simulink model "SM_Offshore_Windturbine"  (R2021a)
settings: Solver=ode4  StartTime=0.0  StopTime=par.sym.Ttot  FixedStep=par.sym.max_dt  MaxStep=par.sym.max_dt  RelTol=1e-3
model workspace: external: MATLAB File C:\Users\d053704\Desktop\MOST\Structure\CAD\CAD_DataFile.m (data not in the file)
undefined symbols (not defined in the file): par, smiData, X, Y, Z
libraries: sm_lib x50, simulink_extras x29, vrlib x18, nesl_utility x10, dspstat3 x9, sharedutil x5, eeGeneralControl x2
(part 2 of 4)

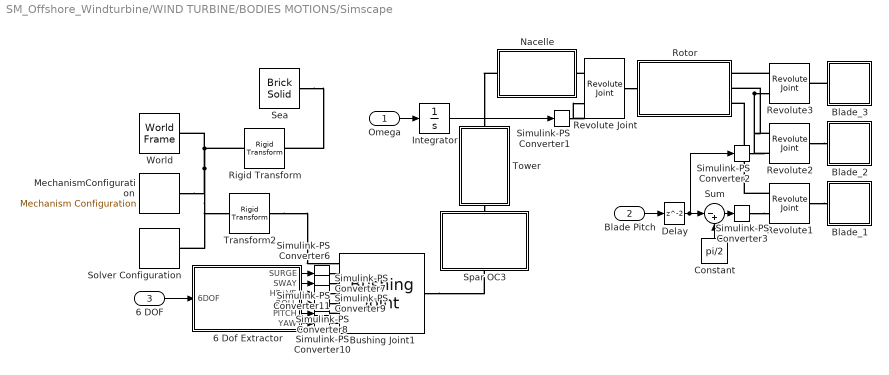
== system SM_Offshore_Windturbine/WIND TURBINE/BODIES MOTIONS/Simscape ==
  Omega : Inport
  Blade Pitch : Inport  Port=2
  6 DOF : Inport  Port=3
  "6 Dof Extractor " : Subsystem
  Blade_1 : Subsystem
  Blade_2 : Subsystem
  Blade_3 : Subsystem
  Bushing Joint1 : sm_lib/Joints/Bushing Joint  JointMode=Normal  SenseConstraintForce=off  SenseConstraintForceX=off  SenseConstraintForceY=off  SenseConstraintForceZ=off  SenseConstraintTorque=off  SenseConstraintTorqueX=off  SenseConstraintTorqueY=off  SenseConstraintTorqueZ=off  SenseTotalForce=off  SenseTotalForceX=off  SenseTotalForceY=off  SenseTotalForceZ=off  SenseTotalTorque=off  SenseTotalTorqueX=off  SenseTotalTorqueY=off  SenseTotalTorqueZ=off  CompositeWrenchDir=FollowerOnBase  CompositeWrenchFrame=BaseFrame  PxEquilibriumPosition=0  PxEquilibriumPositionUnits=m  PxSpringStiffness=0  PxSpringStiffnessUnits=N/m  PxDampingCoefficient=0  PxDampingCoefficientUnits=N/(m/s)  PxTorqueActuationMode=ComputedTorque  PxMotionActuationMode=InputMotion  PxSensePosition=off  PxSenseVelocity=off  PxSenseAcceleration=off  PxSenseTorqueForce=off  PxSenseLowerLimitTorqueForce=off  PxSenseUpperLimitTorqueForce=off  PxLowerLimitSpecify=off  PxLowerLimitBound=-1  PxLowerLimitBoundUnits=m  PxLowerLimitStiffness=1e6  PxLowerLimitStiffnessUnits=N/m  PxLowerLimitDamping=1e3  PxLowerLimitDampingUnits=N/(m/s)  PxLowerLimitTransitionRegionWidth=1e-4  PxLowerLimitTransitionRegionWidthUnits=m  PxUpperLimitSpecify=off  PxUpperLimitBound=1  PxUpperLimitBoundUnits=m  PxUpperLimitStiffness=1e6  PxUpperLimitStiffnessUnits=N/m  PxUpperLimitDamping=1e3  PxUpperLimitDampingUnits=N/(m/s)  PxUpperLimitTransitionRegionWidth=1e-4  PxUpperLimitTransitionRegionWidthUnits=m  PxPositionTargetSpecify=off  PxPositionTargetPriority=High  PxPositionTargetValue=0  PxPositionTargetValueUnits=m  PxVelocityTargetSpecify=off  PxVelocityTargetPriority=High  PxVelocityTargetValue=0  PxVelocityTargetValueUnits=m/s  PyEquilibriumPosition=0  PyEquilibriumPositionUnits=m  PySpringStiffness=0  PySpringStiffnessUnits=N/m  PyDampingCoefficient=0  PyDampingCoefficientUnits=N/(m/s)  PyTorqueActuationMode=ComputedTorque  PyMotionActuationMode=InputMotion  PySensePosition=off  PySenseVelocity=off  PySenseAcceleration=off  PySenseTorqueForce=off  PySenseLowerLimitTorqueForce=off  PySenseUpperLimitTorqueForce=off  PyLowerLimitSpecify=off  PyLowerLimitBound=-1  PyLowerLimitBoundUnits=m  PyLowerLimitStiffness=1e6  PyLowerLimitStiffnessUnits=N/m  PyLowerLimitDamping=1e3  PyLowerLimitDampingUnits=N/(m/s)  PyLowerLimitTransitionRegionWidth=1e-4  PyLowerLimitTransitionRegionWidthUnits=m  PyUpperLimitSpecify=off  PyUpperLimitBound=1  PyUpperLimitBoundUnits=m  PyUpperLimitStiffness=1e6  PyUpperLimitStiffnessUnits=N/m  PyUpperLimitDamping=1e3  PyUpperLimitDampingUnits=N/(m/s)  PyUpperLimitTransitionRegionWidth=1e-4  PyUpperLimitTransitionRegionWidthUnits=m  PyPositionTargetSpecify=off  PyPositionTargetPriority=High  PyPositionTargetValue=0  PyPositionTargetValueUnits=m  PyVelocityTargetSpecify=off  PyVelocityTargetPriority=High  PyVelocityTargetValue=0  PyVelocityTargetValueUnits=m/s  PzEquilibriumPosition=0  PzEquilibriumPositionUnits=m  PzSpringStiffness=0  PzSpringStiffnessUnits=N/m  PzDampingCoefficient=0  PzDampingCoefficientUnits=N/(m/s)  PzTorqueActuationMode=ComputedTorque  PzMotionActuationMode=InputMotion  PzSensePosition=off  PzSenseVelocity=off  PzSenseAcceleration=off  PzSenseTorqueForce=off  PzSenseLowerLimitTorqueForce=off  PzSenseUpperLimitTorqueForce=off  PzLowerLimitSpecify=off  PzLowerLimitBound=-1  PzLowerLimitBoundUnits=m  PzLowerLimitStiffness=1e6  PzLowerLimitStiffnessUnits=N/m  PzLowerLimitDamping=1e3  PzLowerLimitDampingUnits=N/(m/s)  PzLowerLimitTransitionRegionWidth=1e-4  PzLowerLimitTransitionRegionWidthUnits=m  PzUpperLimitSpecify=off  PzUpperLimitBound=1  PzUpperLimitBoundUnits=m  PzUpperLimitStiffness=1e6  PzUpperLimitStiffnessUnits=N/m  PzUpperLimitDamping=1e3  PzUpperLimitDampingUnits=N/(m/s)  PzUpperLimitTransitionRegionWidth=1e-4  PzUpperLimitTransitionRegionWidthUnits=m  PzPositionTargetSpecify=off  PzPositionTargetPriority=High  PzPositionTargetValue=0  PzPositionTargetValueUnits=m  PzVelocityTargetSpecify=off  PzVelocityTargetPriority=High  PzVelocityTargetValue=0  PzVelocityTargetValueUnits=m/s  RxEquilibriumPosition=0  RxEquilibriumPositionUnits=deg  RxSpringStiffness=0  RxSpringStiffnessUnits=N*m/deg  RxDampingCoefficient=0  RxDampingCoefficientUnits=N*m/(deg/s)  RxTorqueActuationMode=ComputedTorque  RxMotionActuationMode=InputMotion  RxSensePosition=off  RxSenseVelocity=off  RxSenseAcceleration=off  RxSenseTorqueForce=off  RxSenseLowerLimitTorqueForce=off  RxSenseUpperLimitTorqueForce=off  RxLowerLimitSpecify=off  RxLowerLimitBound=-90  RxLowerLimitBoundUnits=deg  RxLowerLimitStiffness=1e4  RxLowerLimitStiffnessUnits=N*m/deg  RxLowerLimitDamping=10  RxLowerLimitDampingUnits=N*m/(deg/s)  RxLowerLimitTransitionRegionWidth=0.1  RxLowerLimitTransitionRegionWidthUnits=deg  RxUpperLimitSpecify=off  RxUpperLimitBound=90  RxUpperLimitBoundUnits=deg  RxUpperLimitStiffness=1e4  RxUpperLimitStiffnessUnits=N*m/deg  RxUpperLimitDamping=10  RxUpperLimitDampingUnits=N*m/(deg/s)  RxUpperLimitTransitionRegionWidth=0.1  RxUpperLimitTransitionRegionWidthUnits=deg  RxPositionTargetSpecify=off  RxPositionTargetPriority=High  RxPositionTargetValue=0  RxPositionTargetValueUnits=deg  RxVelocityTargetSpecify=off  RxVelocityTargetPriority=High  RxVelocityTargetValue=0  RxVelocityTargetValueUnits=deg/s  RyEquilibriumPosition=0  RyEquilibriumPositionUnits=deg  RySpringStiffness=0  RySpringStiffnessUnits=N*m/deg  RyDampingCoefficient=0  RyDampingCoefficientUnits=N*m/(deg/s)  RyTorqueActuationMode=ComputedTorque  RyMotionActuationMode=InputMotion  RySensePosition=off  RySenseVelocity=off  RySenseAcceleration=off  RySenseTorqueForce=off  RySenseLowerLimitTorqueForce=off  RySenseUpperLimitTorqueForce=off  RyLowerLimitSpecify=off  RyLowerLimitBound=-90  RyLowerLimitBoundUnits=deg  RyLowerLimitStiffness=1e4  RyLowerLimitStiffnessUnits=N*m/deg  RyLowerLimitDamping=10  RyLowerLimitDampingUnits=N*m/(deg/s)  RyLowerLimitTransitionRegionWidth=0.1  RyLowerLimitTransitionRegionWidthUnits=deg  RyUpperLimitSpecify=off  RyUpperLimitBound=90  RyUpperLimitBoundUnits=deg  RyUpperLimitStiffness=1e4  RyUpperLimitStiffnessUnits=N*m/deg  RyUpperLimitDamping=10  RyUpperLimitDampingUnits=N*m/(deg/s)  RyUpperLimitTransitionRegionWidth=0.1  RyUpperLimitTransitionRegionWidthUnits=deg  RyPositionTargetSpecify=off  RyPositionTargetPriority=High  RyPositionTargetValue=0  RyPositionTargetValueUnits=deg  RyVelocityTargetSpecify=off  RyVelocityTargetPriority=High  RyVelocityTargetValue=0  RyVelocityTargetValueUnits=deg/s  RzEquilibriumPosition=0  RzEquilibriumPositionUnits=deg  RzSpringStiffness=0  RzSpringStiffnessUnits=N*m/deg  RzDampingCoefficient=0  RzDampingCoefficientUnits=N*m/(deg/s)  RzTorqueActuationMode=ComputedTorque  RzMotionActuationMode=InputMotion  RzSensePosition=off  RzSenseVelocity=off  RzSenseAcceleration=off  RzSenseTorqueForce=off  RzSenseLowerLimitTorqueForce=off  RzSenseUpperLimitTorqueForce=off  RzLowerLimitSpecify=off  RzLowerLimitBound=-90  RzLowerLimitBoundUnits=deg  RzLowerLimitStiffness=1e4  RzLowerLimitStiffnessUnits=N*m/deg  RzLowerLimitDamping=10  RzLowerLimitDampingUnits=N*m/(deg/s)  RzLowerLimitTransitionRegionWidth=0.1  RzLowerLimitTransitionRegionWidthUnits=deg  RzUpperLimitSpecify=off  RzUpperLimitBound=90  RzUpperLimitBoundUnits=deg  RzUpperLimitStiffness=1e4  RzUpperLimitStiffnessUnits=N*m/deg  RzUpperLimitDamping=10  RzUpperLimitDampingUnits=N*m/(deg/s)  RzUpperLimitTransitionRegionWidth=0.1  RzUpperLimitTransitionRegionWidthUnits=deg  RzPositionTargetSpecify=off  RzPositionTargetPriority=High  RzPositionTargetValue=0  RzPositionTargetValueUnits=deg  RzVelocityTargetSpecify=off  RzVelocityTargetPriority=High  RzVelocityTargetValue=0  RzVelocityTargetValueUnits=deg/s
  Constant : Constant  Value=pi/2
  Delay : Delay
  Integrator : Integrator
  MechanismConfiguration : sm_lib/Utilities/Mechanism Configuration  UniformGravity=Constant  GravityVector=[0 -9.80665 0]  GravityVectorUnits=m/s^2  GravityUnits=m/s^2  LinearizationDelta=0.001  JointModeTransitionNonlinearIterations=2
  Nacelle : Subsystem
  Revolute Joint : sm_lib/Joints/Revolute Joint  JointMode=Normal  SenseConstraintForce=off  SenseConstraintForceX=off  SenseConstraintForceY=off  SenseConstraintForceZ=off  SenseConstraintTorque=off  SenseConstraintTorqueX=off  SenseConstraintTorqueY=off  SenseConstraintTorqueZ=off  SenseTotalForce=off  SenseTotalForceX=off  SenseTotalForceY=off  SenseTotalForceZ=off  SenseTotalTorque=off  SenseTotalTorqueX=off  SenseTotalTorqueY=off  SenseTotalTorqueZ=off  CompositeWrenchDir=FollowerOnBase  CompositeWrenchFrame=BaseFrame  EquilibriumPosition=0  EquilibriumPositionUnits=deg  SpringStiffness=0  SpringStiffnessUnits=N*m/deg  DampingCoefficient=0  DampingCoefficientUnits=N*m/(rad/s)  TorqueActuationMode=ComputedTorque  MotionActuationMode=InputMotion  SensePosition=off  SenseVelocity=off  SenseAcceleration=off  SenseTorqueForce=off  SenseLowerLimitTorqueForce=off  SenseUpperLimitTorqueForce=off  LowerLimitSpecify=off  LowerLimitBound=-90  LowerLimitBoundUnits=deg  LowerLimitStiffness=1e4  LowerLimitStiffnessUnits=N*m/deg  LowerLimitDamping=10  LowerLimitDampingUnits=N*m/(deg/s)  LowerLimitTransitionRegionWidth=0.1  LowerLimitTransitionRegionWidthUnits=deg  UpperLimitSpecify=off  UpperLimitBound=90  UpperLimitBoundUnits=deg  UpperLimitStiffness=1e4  UpperLimitStiffnessUnits=N*m/deg  UpperLimitDamping=10  UpperLimitDampingUnits=N*m/(deg/s)  UpperLimitTransitionRegionWidth=0.1  UpperLimitTransitionRegionWidthUnits=deg  PositionTargetSpecify=on  PositionTargetPriority=High  PositionTargetValue=0  PositionTargetValueUnits=deg  VelocityTargetSpecify=on  VelocityTargetPriority=High  VelocityTargetValue=12.1/60  VelocityTargetValueUnits=rev/s
  Revolute1 : sm_lib/Joints/Revolute Joint  JointMode=Normal  SenseConstraintForce=off  SenseConstraintForceX=off  SenseConstraintForceY=off  SenseConstraintForceZ=off  SenseConstraintTorque=off  SenseConstraintTorqueX=off  SenseConstraintTorqueY=off  SenseConstraintTorqueZ=off  SenseTotalForce=off  SenseTotalForceX=off  SenseTotalForceY=off  SenseTotalForceZ=off  SenseTotalTorque=off  SenseTotalTorqueX=off  SenseTotalTorqueY=off  SenseTotalTorqueZ=off  CompositeWrenchDir=FollowerOnBase  CompositeWrenchFrame=BaseFrame  EquilibriumPosition=0  EquilibriumPositionUnits=rad  SpringStiffness=0  SpringStiffnessUnits=N*m/rad  DampingCoefficient=0  DampingCoefficientUnits=N*m/(rad/s)  TorqueActuationMode=ComputedTorque  MotionActuationMode=InputMotion  SensePosition=off  SenseVelocity=off  SenseAcceleration=off  SenseTorqueForce=off  SenseLowerLimitTorqueForce=off  SenseUpperLimitTorqueForce=off  LowerLimitSpecify=off  LowerLimitBound=-90  LowerLimitBoundUnits=deg  LowerLimitStiffness=1e4  LowerLimitStiffnessUnits=N*m/deg  LowerLimitDamping=10  LowerLimitDampingUnits=N*m/(deg/s)  LowerLimitTransitionRegionWidth=0.1  LowerLimitTransitionRegionWidthUnits=deg  UpperLimitSpecify=off  UpperLimitBound=90  UpperLimitBoundUnits=deg  UpperLimitStiffness=1e4  UpperLimitStiffnessUnits=N*m/deg  UpperLimitDamping=10  UpperLimitDampingUnits=N*m/(deg/s)  UpperLimitTransitionRegionWidth=0.1  UpperLimitTransitionRegionWidthUnits=deg  PositionTargetSpecify=on  PositionTargetPriority=High  PositionTargetValue=90  PositionTargetValueUnits=deg  VelocityTargetSpecify=off  VelocityTargetPriority=High  VelocityTargetValue=0  VelocityTargetValueUnits=deg/s
  Revolute2 : sm_lib/Joints/Revolute Joint  JointMode=Normal  SenseConstraintForce=off  SenseConstraintForceX=off  SenseConstraintForceY=off  SenseConstraintForceZ=off  SenseConstraintTorque=off  SenseConstraintTorqueX=off  SenseConstraintTorqueY=off  SenseConstraintTorqueZ=off  SenseTotalForce=off  SenseTotalForceX=off  SenseTotalForceY=off  SenseTotalForceZ=off  SenseTotalTorque=off  SenseTotalTorqueX=off  SenseTotalTorqueY=off  SenseTotalTorqueZ=off  CompositeWrenchDir=FollowerOnBase  CompositeWrenchFrame=BaseFrame  EquilibriumPosition=0  EquilibriumPositionUnits=rad  SpringStiffness=0  SpringStiffnessUnits=N*m/rad  DampingCoefficient=0  DampingCoefficientUnits=N*m/(rad/s)  TorqueActuationMode=ComputedTorque  MotionActuationMode=InputMotion  SensePosition=off  SenseVelocity=off  SenseAcceleration=off  SenseTorqueForce=off  SenseLowerLimitTorqueForce=off  SenseUpperLimitTorqueForce=off  LowerLimitSpecify=off  LowerLimitBound=-90  LowerLimitBoundUnits=deg  LowerLimitStiffness=1e4  LowerLimitStiffnessUnits=N*m/deg  LowerLimitDamping=10  LowerLimitDampingUnits=N*m/(deg/s)  LowerLimitTransitionRegionWidth=0.1  LowerLimitTransitionRegionWidthUnits=deg  UpperLimitSpecify=off  UpperLimitBound=90  UpperLimitBoundUnits=deg  UpperLimitStiffness=1e4  UpperLimitStiffnessUnits=N*m/deg  UpperLimitDamping=10  UpperLimitDampingUnits=N*m/(deg/s)  UpperLimitTransitionRegionWidth=0.1  UpperLimitTransitionRegionWidthUnits=deg  PositionTargetSpecify=on  PositionTargetPriority=High  PositionTargetValue=0  PositionTargetValueUnits=deg  VelocityTargetSpecify=off  VelocityTargetPriority=High  VelocityTargetValue=0  VelocityTargetValueUnits=deg/s
  Revolute3 : sm_lib/Joints/Revolute Joint  JointMode=Normal  SenseConstraintForce=off  SenseConstraintForceX=off  SenseConstraintForceY=off  SenseConstraintForceZ=off  SenseConstraintTorque=off  SenseConstraintTorqueX=off  SenseConstraintTorqueY=off  SenseConstraintTorqueZ=off  SenseTotalForce=off  SenseTotalForceX=off  SenseTotalForceY=off  SenseTotalForceZ=off  SenseTotalTorque=off  SenseTotalTorqueX=off  SenseTotalTorqueY=off  SenseTotalTorqueZ=off  CompositeWrenchDir=FollowerOnBase  CompositeWrenchFrame=BaseFrame  EquilibriumPosition=0  EquilibriumPositionUnits=rad  SpringStiffness=0  SpringStiffnessUnits=N*m/rad  DampingCoefficient=0  DampingCoefficientUnits=N*m/(rad/s)  TorqueActuationMode=ComputedTorque  MotionActuationMode=InputMotion  SensePosition=off  SenseVelocity=off  SenseAcceleration=off  SenseTorqueForce=off  SenseLowerLimitTorqueForce=off  SenseUpperLimitTorqueForce=off  LowerLimitSpecify=off  LowerLimitBound=-90  LowerLimitBoundUnits=deg  LowerLimitStiffness=1e4  LowerLimitStiffnessUnits=N*m/deg  LowerLimitDamping=10  LowerLimitDampingUnits=N*m/(deg/s)  LowerLimitTransitionRegionWidth=0.1  LowerLimitTransitionRegionWidthUnits=deg  UpperLimitSpecify=off  UpperLimitBound=90  UpperLimitBoundUnits=deg  UpperLimitStiffness=1e4  UpperLimitStiffnessUnits=N*m/deg  UpperLimitDamping=10  UpperLimitDampingUnits=N*m/(deg/s)  UpperLimitTransitionRegionWidth=0.1  UpperLimitTransitionRegionWidthUnits=deg  PositionTargetSpecify=on  PositionTargetPriority=High  PositionTargetValue=0  PositionTargetValueUnits=deg  VelocityTargetSpecify=off  VelocityTargetPriority=High  VelocityTargetValue=0  VelocityTargetValueUnits=deg/s
  Rigid Transform : sm_lib/Frames and Transforms/Rigid Transform  TranslationMethod=Cartesian  TranslationStandardOffset=0  TranslationLengthUnit=m  TranslationStandardAxis=+Z  TranslationCartesianOffset=[-5 5 2]  TranslationROffset=0  TranslationROffsetUnits=m  TranslationZOffset=0  TranslationZOffsetUnits=m  TranslationThetaOffset=0  TranslationThetaOffsetUnits=deg  RotationMethod=None  RotationAngleUnits=deg  RotationStandardAxis=+Z  RotationAngle=0.0  RotationArbitraryAxis=[0 0 1]  FollAlignAxisA=+X  BaseAlignAxisA=+Y  FollAlignAxisB=+Y  BaseAlignAxisB=+Z  RotationSequenceAxes=FollowerAxes  RotationSequence=XYX  RotationSequenceAngles=[0 0 0]  RotationSequenceAnglesUnits=deg  RotationMatrix=[1 0 0; 0 1 0; 0 0 1]
  Rotor : Subsystem
  Sea : sm_lib/Body Elements/Brick Solid  GraphicAmbientColor=[0.15 0.15 0.15 1.0]  BasedOnType=Density  BrickDimensions=[300 300 1]  BrickDimensionUnits=m  CenterOfMass=[0 0 0]  CenterOfMassUnits=m  GraphicDiffuseColor=[0.0 0.79607844 1.0]  Density=1000  DensityUnits=kg/m^3  DoExposeReferenceFrame=on  GraphicEmissiveColor=[0.0 0.0 0.0 1.0]  ExportEntireGeometry=off  SerializedFrames=<Frames/>  MarkerShape=Sphere  MarkerSize=10  GraphicType=FromGeometry  InertiaType=CalculateFromGeometry  Mass=1  MassUnits=kg  MomentsOfInertia=[1 1 1]  MomentsOfInertiaUnits=kg*m^2  GraphicOpacity=0.5  ProductsOfInertia=[0 0 0]  ProductsOfInertiaUnits=kg*m^2  GraphicShininess=75  GraphicSpecularColor=[0.5 0.5 0.5 1.0]  GraphicVisPropType=SimpleVisualProperties
  Simulink-PS Converter{1..3,6..11} (9 alike) : nesl_utility/Simulink-PS Converter  PhysicalDomain=network_engine_domain  SubClassName=ps_input  LeftPortType=input  RightPortType=output  PseudoPeriodic=off  Frequencies=[]  NoiseDistribution=none  NoiseParameters=[]  Unit=1  AffineConversion=off  FilteringAndDerivatives=filter  SimscapeFilterOrder=2  InputFilterTimeConstant=0.05  UdotUserProvided=0
      settings: SourceProductBaseCode=PW,SS
  Solver Configuration : nesl_utility/Solver Configuration  PhysicalDomain=network_engine_domain  SubClassName=solver  LeftPortType=input  RightPortType=generic  Tones=[]  Harmonics=[]  SimulateNoise=off  Profile=off  UseLocalSampling=off  EnableSwitchedLinearOptims=on  FrequencyDomain=off  UseCCode=off  RelTol=0.001  AbsTol=1e-06  MinStep=1e-09  ToWorkspace=off  RevertToSquareIcSolve=off  NumHomotopyIterations=100  PhasorMode=off  PhasorModeNumHarmonics=1  DoDC=off  ResidualTolerance=1e-09  UseLocalSolver=off  LocalSolverChoice=NE_BACKWARD_EULER_ADVANCER  LocalSolverSampleTime=0.001  DoFixedCost=off  MaxNonlinIter=3  MaxModeIter=2  ComputeImpulses=off  ImpulseIterations=2  LinearAlgebra=auto  EquationFormulation=NE_TIME_EF  DelaysMemoryBudget=1024  AutomaticFiltering=on  FilteringTimeConstant=0.001  PartitionStorageMethod=AS_NEEDED  PartitionMemoryBudget=1024  PartitionMethod=FAST
      settings: SourceProductBaseCode=PW,SS
  Spar OC3 : Subsystem
  Sum : Sum  Inputs=|-+
  Tower : Subsystem
  Transform2 : sm_lib/Frames and Transforms/Rigid Transform  TranslationMethod=Cartesian  TranslationStandardOffset=0  TranslationLengthUnit=m  TranslationStandardAxis=+Z  TranslationCartesianOffset=smiData.RigidTransform(17).translation  TranslationROffset=0  TranslationROffsetUnits=m  TranslationZOffset=0  TranslationZOffsetUnits=m  TranslationThetaOffset=0  TranslationThetaOffsetUnits=deg  RotationMethod=ArbitraryAxis  RotationAngleUnits=rad  RotationStandardAxis=+Z  RotationAngle=smiData.RigidTransform(17).angle  RotationArbitraryAxis=smiData.RigidTransform(17).axis  FollAlignAxisA=+X  BaseAlignAxisA=+Y  FollAlignAxisB=+Y  BaseAlignAxisB=+Z  RotationSequenceAxes=FollowerAxes  RotationSequence=XYX  RotationSequenceAngles=[0 0 0]  RotationSequenceAnglesUnits=deg  RotationMatrix=[1 0 0; 0 1 0; 0 0 1]
  World : sm_lib/Frames and Transforms/World Frame
  wires:
  Integrator/1 -> Simulink-PS Converter1/1
  Blade Pitch/1 -> Delay/1
  "6 Dof Extractor "/1(SURGE) -> Simulink-PS Converter6/1
  "6 Dof Extractor "/6(YAW) -> Simulink-PS Converter11/1
  Sum/1 -> Simulink-PS Converter3/1
  Constant/1 -> Sum/2
  "6 Dof Extractor "/3(HEAVE) -> Simulink-PS Converter8/1
  "6 Dof Extractor "/5(PITCH) -> Simulink-PS Converter10/1
  "6 Dof Extractor "/4(ROLL) -> Simulink-PS Converter9/1
  6 DOF/1 -> "6 Dof Extractor "/1(6DOF)
  "6 Dof Extractor "/2(SWAY) -> Simulink-PS Converter7/1
  Delay/1 -> Simulink-PS Converter2/1, Sum/1
  Omega/1 -> Integrator/1
  connections:
  Revolute2/LConn1 -- Rotor/RConn2
  Simulink-PS Converter8/RConn1 -- Bushing Joint1/LConn4
  Revolute1/LConn1 -- Rotor/RConn3
  Simulink-PS Converter7/RConn1 -- Bushing Joint1/LConn3
  Nacelle/LConn1 -- Tower/RConn1
  Revolute2/RConn1 -- Blade_2/LConn1
  Simulink-PS Converter3/RConn1 -- Revolute1/LConn2
  Revolute Joint/LConn1 -- Nacelle/RConn1
  Revolute Joint/RConn1 -- Rotor/LConn1
  Transform2/RConn1 -- Bushing Joint1/LConn1
  Bushing Joint1/LConn6 -- Simulink-PS Converter10/RConn1
  Bushing Joint1/LConn7 -- Simulink-PS Converter11/RConn1
  Simulink-PS Converter6/RConn1 -- Bushing Joint1/LConn2
  Bushing Joint1/RConn1 -- Spar OC3/LConn1
  Revolute1/RConn1 -- Blade_1/LConn1
  Rigid Transform/LConn1 -- World/RConn1 -- MechanismConfiguration/RConn1 -- Solver Configuration/RConn1 -- Transform2/LConn1
  Simulink-PS Converter9/RConn1 -- Bushing Joint1/LConn5
  Revolute3/LConn1 -- Rotor/RConn1
  Simulink-PS Converter1/RConn1 -- Revolute Joint/LConn2
  Blade_3/LConn1 -- Revolute3/RConn1
  Revolute3/LConn2 -- Simulink-PS Converter2/RConn1 -- Revolute2/LConn2
  Tower/LConn1 -- Spar OC3/RConn1
  Sea/RConn1 -- Rigid Transform/RConn1

== system SM_Offshore_Windturbine/WIND TURBINE/CONTROL SYSTEM/BLADE PITCH CONTROL ==
  note: GK(theta)
  note: PITCH CONTROL
  Filtered generator speed : Inport
  Constant2 : Constant
  Constant3 : Constant
  Divide : Product  Inputs=*/
  Divide1 : Product  Inputs=*/
  Gain : Gain  Gain=pi/2
  Gain1 : Gain  Gain=par.WT.ctrl.PITCH.Kp_c
  Gain2 : Gain  Gain=par.WT.ctrl.PITCH.Ki_c
  Integrator Limited : Integrator  InitialCondition=par.IC.BlPtc0/180*pi / (par.WT.ctrl.PITCH.Ki_c / (1 + par.IC.BlPtc0/par.WT.ctrl.PITCH.thetak))  LimitOutput=on  LowerSaturationLimit=0
  Max : MinMax  Function=max  Inputs=2
  Memory : Memory  InitialCondition=par.IC.BlPtc0
  Min : MinMax  Inputs=2
  Pitch rate limiter : RateLimiter  RisingSlewLimit=par.WT.ctrl.PITCH.ratelim/180*pi  FallingSlewLimit=-par.WT.ctrl.PITCH.ratelim/180*pi  SampleTimeMode=inherited
  Pitch saturation : Saturate  UpperLimit=pi/2  LowerLimit=0
  Product : Product  RndMeth=Zero
  Product1 : Product  RndMeth=Zero
  Radians to Degrees : simulink_extras/Transformations/Radians to Degrees
  Radians to Degrees3 : simulink_extras/Transformations/Radians to Degrees
  Reciprocal : Product  Inputs=/
  Rotor nominal speed : Constant  Value=par.WT.ctrl.PTO.wnom*pi/30
  Sum : Sum  Inputs=+-|
  Sum1 : Sum  Inputs=|++
  Sum2 : Sum
  Theta_k : Constant  Value=par.WT.ctrl.PITCH.thetak
  Zero : Constant  Value=0
  Blade pitch : Outport  VectorParamsAs1DForOutWhenUnconnected=off
  tag scope: BlPITCH=global
  wires:
  Pitch saturation/1 -> Pitch rate limiter/1  "Blade pitch"
  Gain/1 -> Min/2
  Radians to Degrees3/1 -> Memory/1  "BlPitch"
  Zero/1 -> Max/1
  Max/1 -> Min/1
  Radians to Degrees/1 -> [BlPITCH]  "BlPitch"
  Divide/1 -> Sum1/1
  Memory/1 -> Divide/1
  Constant2/1 -> Sum1/2
  Min/1 -> Product1/1
  Reciprocal/1 -> Gain/1
  Theta_k/1 -> Divide/2
  Sum1/1 -> Divide1/2
  Sum2/1 -> Pitch saturation/1
  Constant3/1 -> Divide1/1
  Sum/1 -> Product/1, Integrator Limited/1  "Generator speed error"
  Product/1 -> Sum2/1
  Divide1/1 -> Gain2/1, Gain1/1
  Pitch rate limiter/1 -> Radians to Degrees3/1, Blade pitch/1, Radians to Degrees/1  "Blade pitch"
  Gain1/1 -> Product/2  "Kp"
  Product1/1 -> Sum2/2
  Gain2/1 -> Reciprocal/1, Product1/2  "Ki"
  Rotor nominal speed/1 -> Sum/2
  Integrator Limited/1 -> Max/2
  Filtered generator speed/1 -> Sum/1

== system SM_Offshore_Windturbine/WIND TURBINE/CONTROL SYSTEM/TORQUE CONTROL ==
  note: GENERATOR-TORQUE CONTROL
  Filtered generator speed : Inport
  Blade Pitch : Inport  Port=2
  Blade Pitch min for const Power law : Constant  Value=par.WT.ctrl.PITCH.BlPtch_min
  Brake dynamics : TransferFcn  Denominator=[par.WT.ctrl.PTO.GENBRK_tau 1]
  Brake hysteresis : Relay  OnSwitchValue=par.WT.ctrl.PTO.GENBRK_lim_on  OffSwitchValue=par.WT.ctrl.PTO.GENBRK_lim_off  OnOutputValue=par.WT.ctrl.PTO.GENBRK
  Constant Power Law : Subsystem  TreatAsAtomicUnit=on
  Constant Torque Law : Subsystem  TreatAsAtomicUnit=on
  Control torque law : Lookup_n-D  NumberOfTableDimensions=1  BreakpointsForDimension1=par.WT.ctrl.PTO.GENSPEED  Table=par.WT.ctrl.PTO.GENTRQ  RndMeth=Simplest  InputSameDT=on
  If : If  NumInputs=2  IfExpression=u1 > u2
  Merge : Merge
  Radians to Degrees3 : simulink_extras/Transformations/Radians to Degrees
  Sum3 : Sum  Inputs=++|
  Torque rate limiter : RateLimiter  RisingSlewLimit=par.WT.ctrl.PTO.ratelim  FallingSlewLimit=-par.WT.ctrl.PTO.ratelim  SampleTimeMode=inherited
  rads2rpm : Gain  Gain=30/pi
  Generator torque : Outport  VectorParamsAs1DForOutWhenUnconnected=off
  tag scope: GENSPD=global, GENTRQ=global
  wires:
  Control torque law/1 -> Constant Torque Law/1(BlPtch=0)
  Radians to Degrees3/1 -> If/1
  If/2 -> Constant Torque Law/Action
  Blade Pitch min for const Power law/1 -> If/2
  Filtered generator speed/1 -> rads2rpm/1, Constant Power Law/1(BlPtch>0)
  Constant Power Law/1(" ") -> Merge/1
  Torque rate limiter/1 -> Sum3/2, [GENTRQ]
  Brake hysteresis/1 -> Brake dynamics/1
  Sum3/1 -> Generator torque/1  "Generator torque"
  Brake dynamics/1 -> Sum3/1
  Constant Torque Law/1(" ") -> Merge/2
  If/1 -> Constant Power Law/Action
  Merge/1 -> Torque rate limiter/1
  rads2rpm/1 -> Control torque law/1, [GENSPD], Brake hysteresis/1
  Blade Pitch/1 -> Radians to Degrees3/1

== system SM_Offshore_Windturbine/WIND TURBINE/ROTOR LOADS/Aerodynamic Loads ==
  6 DOF : Inport
  Azimuth : Inport  Port=2
  Omega : Inport  Port=3
  blade pitch : Inport  Port=4
  Atan : Trigonometry  Operator=atan
  Blade 1 : Subsystem
  Blade 2 : Subsystem
  Blade 3 : Subsystem
  Clock : Clock
      settings: Decimation=20
  Constant1 : Constant  Value=par.WT.BEM.zNods
  Degrees to Radians : simulink_extras/Transformations/Degrees to Radians
  Divide : Product  Inputs=*/
  Integration : MATLAB Function  TreatAsAtomicUnit=on
  Selector : Selector  InputPortWidth=3  IndexOptions=Index vector (dialog)  Indices=1  OutputSizes=1
  Selector1 : Selector  InputPortWidth=3  IndexOptions=Index vector (dialog)  Indices=2  OutputSizes=1
  Skew correction 1 : ModelReference  ModelNameDialog=Skew_correction_1.slxp  ModelReferenceVersion=5.18  CopyOfModelProtected=on
  Skew correction 2 : ModelReference  ModelNameDialog=Skew_correction_1.slxp  ModelReferenceVersion=5.18  CopyOfModelProtected=on
  Skew correction 3 : ModelReference  ModelNameDialog=Skew_correction_1.slxp  ModelReferenceVersion=5.18  CopyOfModelProtected=on
  Sum : Sum  Inputs=+++
  Wind Direct : Outport  VectorParamsAs1DForOutWhenUnconnected=off
  RotorTorque : Outport  Port=2  VectorParamsAs1DForOutWhenUnconnected=off
  AeroLoads : Outport  Port=3  VectorParamsAs1DForOutWhenUnconnected=off
  wires:
  Blade 1/3(Azimuth1) -> Skew correction 1/4
  Integration/1(RotTrq) -> RotorTorque/1
  Omega/1 -> Blade 3/2(Omega), Blade 2/2(Omega), Blade 1/2(Omega)
  6 DOF/1 -> Blade 3/4(6 DOF), Blade 2/4(6 DOF), Blade 1/4(6 DOF)
  blade pitch/1 -> Blade 3/3(blade pitch), Blade 2/3(blade pitch), Blade 1/3(blade pitch)
  Constant1/1 -> Skew correction 1/1, Integration/2(zNods), Skew correction 3/1, Skew correction 2/1
  Clock/1 -> Blade 3/5(Time), Blade 2/5(Time), Blade 1/5(Time)
  Blade 1/1(AIF) -> Skew correction 1/2
  Blade 1/2(TIF) -> Skew correction 1/3
  Blade 1/4(Cn) -> Skew correction 1/5
  Blade 1/5(Ct) -> Skew correction 1/6
  Blade 1/6(Vx) -> Skew correction 1/7
  Blade 1/7(Vy) -> Skew correction 1/8
  Blade 2/1(AIF) -> Skew correction 2/2
  Blade 2/2(TIF) -> Skew correction 2/3
  Blade 2/3(Azimuth2) -> Skew correction 2/4
  Blade 2/4(Cn) -> Skew correction 2/5
  Blade 2/5(Ct) -> Skew correction 2/6
  Blade 2/6(Vx) -> Skew correction 2/7
  Blade 2/7(Vy) -> Skew correction 2/8
  Blade 3/1(AIF) -> Skew correction 3/2
  Blade 3/2(TIF) -> Skew correction 3/3
  Blade 3/3(Azimuth3) -> Skew correction 3/4
  Blade 3/4(Cn) -> Skew correction 3/5
  Blade 3/5(Ct) -> Skew correction 3/6
  Blade 3/6(Vx) -> Skew correction 3/7
  Blade 3/7(Vy) -> Skew correction 3/8
  Blade 2/8(V0) -> Sum/2
  Blade 1/8(V0) -> Sum/1
  Blade 3/8(V0) -> Sum/3
  Sum/1 -> Skew correction 2/9, Skew correction 1/9, Skew correction 3/9, Selector/1, Selector1/1
  Azimuth/1 -> Degrees to Radians/1, Blade 3/1(Azimuth), Blade 2/1(Azimuth), Blade 1/1(Azimuth)
  Skew correction 3/2 -> Integration/8(pT3)
  Skew correction 3/1 -> Integration/7(pN3)
  Skew correction 2/2 -> Integration/6(pT2)
  Skew correction 2/1 -> Integration/5(pN2)
  Skew correction 1/2 -> Integration/4(pT1)
  Skew correction 1/1 -> Integration/3(pN1)
  Degrees to Radians/1 -> Integration/1(Azimuth)
  Integration/2(AeroLoads) -> AeroLoads/1
  Selector1/1 -> Divide/1
  Selector/1 -> Divide/2
  Divide/1 -> Atan/1
  Atan/1 -> Wind Direct/1

== system SM_Offshore_Windturbine/WIND TURBINE/ROTOR LOADS/Omega to Azimuth ==
  Rotor speed : Inport
  Floor : Rounding
  Gain3 : Gain  Gain=1/(2*pi)
  Gain4 : Gain  Gain=360
  Integrator : Integrator
  Sum2 : Sum  Inputs=|-+
  Out1 : Outport  VectorParamsAs1DForOutWhenUnconnected=off
  tag scope: Azimuth=global
  wires:
  Gain4/1 -> [Azimuth], Out1/1
  Sum2/1 -> Gain4/1
  Floor/1 -> Sum2/1
  Integrator/1 -> Gain3/1
  Gain3/1 -> Sum2/2, Floor/1
  Rotor speed/1 -> Integrator/1

== system SM_Offshore_Windturbine/WIND TURBINE/ROTOR LOADS/TowerBaseLoads ==
  6 DOF : Inport
  AeroLoads : Inport  Port=2
  Control torque : Inport  Port=3
  3D rotation matrix : Subsystem
  Constant : Constant  Value=[0 0 89.57]
  Constant2 : Constant  Value=(par.WT.prop.dtweight+par.WT.prop.towerweight)*9.80665
  Cross Product : vrlib/Utilities/Cross Product
  Demux : Demux  Outputs=3
  Demux1 : Demux  Outputs=3
  Matrix Multiply : Product  Multiplication=Matrix(*)
  Matrix Multiply1 : Product  Multiplication=Matrix(*)
  Matrix Multiply2 : Product  Multiplication=Matrix(*)
  Mux : Mux  Inputs=2
  Mux1 : Mux  Inputs=2
  Mux2 : Mux  Inputs=3
  Mux3 : Mux  Inputs=3
  Selector : Selector  InputPortWidth=6  IndexOptions=Index vector (dialog)  Indices=[1 2 3]  OutputSizes=1
  Selector3 : Selector  InputPortWidth=6  IndexOptions=Index vector (dialog)  Indices=[5 6]  OutputSizes=1
  Sum : Sum  Inputs=-+|
  Sum1 : Sum
  "rx,ry, rz" : Selector  InputPortWidth=18  IndexOptions=Index vector (dialog)  Indices=[4 5 6]  OutputSizes=1
  WTForces : Outport  VectorParamsAs1DForOutWhenUnconnected=off
  tag scope: ROTTHR=global
  wires:
  AeroLoads/1 -> Selector3/1, Selector/1
  "rx,ry, rz"/1 -> 3D rotation matrix/1(hull_rotation)
  6 DOF/1 -> "rx,ry, rz"/1
  Matrix Multiply/1 -> Demux1/1, Demux/1
  3D rotation matrix/1(R(rx,ry,rz)) -> Matrix Multiply1/1, Matrix Multiply2/1, Matrix Multiply/1
  Constant/1 -> Matrix Multiply2/2
  Demux/1 -> [ROTTHR], Mux3/1
  Demux/2 -> Mux3/2
  Constant2/1 -> Sum/1
  Demux/3 -> Sum/2
  Sum/1 -> Mux3/3
  Matrix Multiply2/1 -> Cross Product/1
  Mux3/1 -> Mux/1
  Matrix Multiply1/1 -> Sum1/2
  Cross Product/1 -> Sum1/1
  Sum1/1 -> Mux/2
  Mux/1 -> WTForces/1
  Mux1/1 -> Matrix Multiply1/2
  Selector3/1 -> Mux1/2
  Control torque/1 -> Mux1/1
  Selector/1 -> Matrix Multiply/2
  Demux1/3 -> Mux2/3
  Demux1/2 -> Mux2/2
  Demux1/1 -> Mux2/1
  Mux2/1 -> Cross Product/2

== system SM_Offshore_Windturbine/HULL/Viscous loads/Subsystem1/3D rotation matrix ==
  hull_rotation : Inport
  Constant : Constant
  Create 3x3 Matrix : sharedutil/Create 3x3 Matrix  aMode=aMode
      settings: SourceProductBaseCode=AE,PW,DR,MT,UV,VE
  Fcn1 : Fcn  Expr=u(2)*u(7) + u(3)*u(1)*(u(8)-1)
  Fcn11 : Fcn  Expr=u(4)*u(8) + u(5) + u(6)
  Fcn2 : Fcn  Expr=-u(2)*u(7) + u(1)*u(3)*(u(8)-1)
  Fcn3 : Fcn  Expr=u(5)*u(8) + u(4) + u(6)
  Fcn4 : Fcn  Expr=-u(1)*u(7) + u(3)*u(2)*(u(8)-1)
  Fcn5 : Fcn  Expr=u(1)*u(7) + u(3)*u(2)*(u(8)-1)
  Fcn7 : Fcn  Expr=u(6)*u(8) + u(4) + u(5)
  Fcn8 : Fcn  Expr=u(3)*u(7) + u(1)*u(2)*(u(8)-1)
  Fcn9 : Fcn  Expr=-u(3)*u(7) + u(1)*u(2)*(u(8)-1)
  If : If  IfExpression=u1 == 0
  If Action Subsystem : Subsystem  TreatAsAtomicUnit=on
  If Action Subsystem1 : Subsystem  TreatAsAtomicUnit=on
  Merge : Merge
  Mux : Mux  Inputs=8
  Sqrt : Sqrt  SaturateOnIntegerOverflow=on
  Sum : Sum  Inputs=+++|
  Sum1 : Sum  Inputs=++|
  TETA1 : Math  Operator=square  SignedPower=on  SaturateOnIntegerOverflow=on
  TETA2 : Math  Operator=square  SignedPower=on  SaturateOnIntegerOverflow=on
  TETA3 : Math  Operator=square  SignedPower=on  SaturateOnIntegerOverflow=on
  teta1 : Selector  InputPortWidth=3  IndexOptions=Index vector (dialog)  Indices=1  OutputSizes=1
  teta2 : Selector  InputPortWidth=3  IndexOptions=Index vector (dialog)  Indices=2  OutputSizes=1
  teta3 : Selector  InputPortWidth=3  IndexOptions=Index vector (dialog)  Indices=3  OutputSizes=1
  R(rx,ry,rz) : Outport  VectorParamsAs1DForOutWhenUnconnected=off
  wires:
  hull_rotation/1 -> teta1/1, teta3/1, teta2/1
  teta1/1 -> Mux/1, TETA1/1
  teta2/1 -> Mux/2, TETA2/1
  teta3/1 -> Mux/3, TETA3/1
  TETA2/1 -> Mux/5, Sum/2
  TETA1/1 -> Mux/4, Sum/1
  TETA3/1 -> Mux/6, Sum/3
  Sum/1 -> Mux/7, Sum1/1, If Action Subsystem1/1(TETA), If/1  "TETA"
  Sum1/1 -> Sqrt/1
  Sqrt/1 -> If Action Subsystem1/2(rad), Mux/8  "rad"
  Fcn4/1 -> Create 3x3 Matrix/6
  Fcn3/1 -> Create 3x3 Matrix/5
  Fcn8/1 -> Create 3x3 Matrix/4
  Fcn2/1 -> Create 3x3 Matrix/7
  Fcn1/1 -> Create 3x3 Matrix/3
  Fcn7/1 -> Create 3x3 Matrix/9
  Fcn11/1 -> Create 3x3 Matrix/1
  Fcn5/1 -> Create 3x3 Matrix/8
  Fcn9/1 -> Create 3x3 Matrix/2
  Mux/1 -> Fcn3/1, Fcn4/1, Fcn2/1, Fcn5/1, Fcn7/1, Fcn8/1, Fcn1/1, Fcn9/1, Fcn11/1
  Constant/1 -> Sum1/2
  If/2 -> If Action Subsystem1/Action
  If Action Subsystem/1(R) -> Merge/2
  Merge/1 -> R(rx,ry,rz)/1
  If/1 -> If Action Subsystem/Action
  If Action Subsystem1/1(R) -> Merge/1
  Create 3x3 Matrix/1 -> If Action Subsystem1/3(T)

== system SM_Offshore_Windturbine/HULL/Viscous loads/Subsystem1/Subsystem ==
  Time : Inport
  Constant : Constant  Value=par.sym.dt
  Constant1 : Constant  Value=par.wave.velocities.VX
  Constant3 : Constant  Value=par.wave.velocities.VY
  Direct Lookup Table (n-D) : LookupNDDirect  InputsSelectThisObjectFromTable=Vector  TableIsInput=on
  Direct Lookup Table (n-D)1 : LookupNDDirect  InputsSelectThisObjectFromTable=Vector  TableIsInput=on
  Divide : Product  Inputs=*/
  Transpose : Math  Operator=transpose  SignedPower=on  SaturateOnIntegerOverflow=on
  Transpose1 : Math  Operator=transpose  SignedPower=on  SaturateOnIntegerOverflow=on
  VxVec : Outport
  VzVec : Outport  Port=2
  wires:
  Transpose/1 -> Direct Lookup Table (n-D)/2
  Constant1/1 -> Transpose/1
  Constant/1 -> Divide/2
  Divide/1 -> Direct Lookup Table (n-D)1/1, Direct Lookup Table (n-D)/1
  Direct Lookup Table (n-D)/1 -> VxVec/1
  Transpose1/1 -> Direct Lookup Table (n-D)1/2
  Constant3/1 -> Transpose1/1
  Time/1 -> Divide/1
  Direct Lookup Table (n-D)1/1 -> VzVec/1

== system SM_Offshore_Windturbine/HULL/Viscous loads/Subsystem1/Wave velocities ==
  hull_rot_speed : Inport
  z_plat : Inport  Port=2
  Zrot : Inport  Port=3
  VxVec : Inport  Port=4
  VyVec : Inport  Port=5
  Mux : Mux  Inputs=10
  Mux1 : Mux  Inputs=10
  Selector : Selector  NumberOfDimensions=2  InputPortWidth=10  IndexOptions=Index vector (dialog),Index vector (dialog)  Indices=[1 2 3],1  OutputSizes=1,1
  Selector1 : Selector  NumberOfDimensions=2  InputPortWidth=10  IndexOptions=Index vector (dialog),Index vector (dialog)  Indices=[1 2 3],2  OutputSizes=1,1
  Selector2 : Selector  NumberOfDimensions=2  InputPortWidth=10  IndexOptions=Index vector (dialog),Index vector (dialog)  Indices=[1 2 3],3  OutputSizes=1,1
  Selector3 : Selector  NumberOfDimensions=2  InputPortWidth=10  IndexOptions=Index vector (dialog),Index vector (dialog)  Indices=[1 2 3],4  OutputSizes=1,1
  Selector4 : Selector  NumberOfDimensions=2  InputPortWidth=10  IndexOptions=Index vector (dialog),Index vector (dialog)  Indices=[1 2 3],5  OutputSizes=1,1
  Selector5 : Selector  NumberOfDimensions=2  InputPortWidth=10  IndexOptions=Index vector (dialog),Index vector (dialog)  Indices=[1 2 3],6  OutputSizes=1,1
  Selector6 : Selector  NumberOfDimensions=2  InputPortWidth=10  IndexOptions=Index vector (dialog),Index vector (dialog)  Indices=[1 2 3],7  OutputSizes=1,1
  Selector7 : Selector  NumberOfDimensions=2  InputPortWidth=10  IndexOptions=Index vector (dialog),Index vector (dialog)  Indices=[1 2 3],8  OutputSizes=1,1
  Selector8 : Selector  NumberOfDimensions=2  InputPortWidth=10  IndexOptions=Index vector (dialog),Index vector (dialog)  Indices=[1 2 3],9  OutputSizes=1,1
  Selector9 : Selector  NumberOfDimensions=2  InputPortWidth=10  IndexOptions=Index vector (dialog),Index vector (dialog)  Indices=[1 2 3],10  OutputSizes=1,1
  Subsystem : Subsystem
  Subsystem1 : Subsystem
  Subsystem2 : Subsystem
  Subsystem3 : Subsystem
  Subsystem4 : Subsystem
  Subsystem5 : Subsystem
  Subsystem6 : Subsystem
  Subsystem7 : Subsystem
  Subsystem8 : Subsystem
  Subsystem9 : Subsystem
  Wavex(n) : Outport  VectorParamsAs1DForOutWhenUnconnected=off
  Wavey(n) : Outport  Port=2  VectorParamsAs1DForOutWhenUnconnected=off
  wires:
  hull_rot_speed/1 -> Subsystem1/1(Hull rot spd), Subsystem2/1(Hull rot spd), Subsystem3/1(Hull rot spd), Subsystem4/1(Hull rot spd), Subsystem5/1(Hull rot spd), Subsystem6/1(Hull rot spd), Subsystem7/1(Hull rot spd), Subsystem9/1(Hull rot spd), Subsystem8/1(Hull rot spd), Subsystem/1(Hull rot spd)
  Zrot/1 -> Selector9/1, Selector8/1, Selector7/1, Selector6/1, Selector5/1, Selector4/1, Selector3/1, Selector2/1, Selector1/1, Selector/1
  VxVec/1 -> Subsystem1/4(VxVec), Subsystem2/4(VxVec), Subsystem3/4(VxVec), Subsystem4/4(VxVec), Subsystem5/4(VxVec), Subsystem6/4(VxVec), Subsystem7/4(VxVec), Subsystem9/4(VxVec), Subsystem8/4(VxVec), Subsystem/4(VxVec)
  z_plat/1 -> Subsystem1/3(Zplat), Subsystem2/3(Zplat), Subsystem3/3(Zplat), Subsystem4/3(Zplat), Subsystem5/3(Zplat), Subsystem6/3(Zplat), Subsystem7/3(Zplat), Subsystem9/3(Zplat), Subsystem8/3(Zplat), Subsystem/3(Zplat)
  VyVec/1 -> Subsystem1/5(VyVec), Subsystem2/5(VyVec), Subsystem3/5(VyVec), Subsystem4/5(VyVec), Subsystem5/5(VyVec), Subsystem6/5(VyVec), Subsystem7/5(VyVec), Subsystem9/5(VyVec), Subsystem8/5(VyVec), Subsystem/5(VyVec)
  Selector/1 -> Subsystem/2(Zrot1)
  Selector1/1 -> Subsystem1/2(Zrot1)
  Selector2/1 -> Subsystem2/2(Zrot1)
  Selector3/1 -> Subsystem3/2(Zrot1)
  Selector4/1 -> Subsystem4/2(Zrot1)
  Selector9/1 -> Subsystem9/2(Zrot1)
  Selector5/1 -> Subsystem5/2(Zrot1)
  Selector6/1 -> Subsystem6/2(Zrot1)
  Selector7/1 -> Subsystem7/2(Zrot1)
  Selector8/1 -> Subsystem8/2(Zrot1)
  Mux/1 -> Wavex(n)/1
  Mux1/1 -> Wavey(n)/1
  Subsystem/1(WaveVx1) -> Mux/1
  Subsystem1/1(WaveVx1) -> Mux/2
  Subsystem2/1(WaveVx1) -> Mux/3
  Subsystem3/1(WaveVx1) -> Mux/4
  Subsystem4/1(WaveVx1) -> Mux/5
  Subsystem5/1(WaveVx1) -> Mux/6
  Subsystem6/1(WaveVx1) -> Mux/7
  Subsystem7/1(WaveVx1) -> Mux/8
  Subsystem8/1(WaveVx1) -> Mux/9
  Subsystem9/1(WaveVx1) -> Mux/10
  Subsystem/2(WaveVy1) -> Mux1/1
  Subsystem1/2(WaveVy1) -> Mux1/2
  Subsystem2/2(WaveVy1) -> Mux1/3
  Subsystem3/2(WaveVy1) -> Mux1/4
  Subsystem4/2(WaveVy1) -> Mux1/5
  Subsystem5/2(WaveVy1) -> Mux1/6
  Subsystem6/2(WaveVy1) -> Mux1/7
  Subsystem7/2(WaveVy1) -> Mux1/8
  Subsystem8/2(WaveVy1) -> Mux1/9
  Subsystem9/2(WaveVy1) -> Mux1/10

== system SM_Offshore_Windturbine/WIND TURBINE/BODIES MOTIONS/Simscape/6 Dof Extractor  ==
  note: PITCH
  note: HEAVE
  note: SURGE
  6DOF : Inport  PortDimensions=18
  rx,rxdot,rxdotdot : Selector  InputPortWidth=18  IndexOptions=Index vector (dialog)  Indices=4  OutputSizes=1
  ry,rydot,rydotdot : Selector  InputPortWidth=18  IndexOptions=Index vector (dialog)  Indices=5  OutputSizes=1
  "rz,rzdot,rzdotdot " : Selector  InputPortWidth=18  IndexOptions=Index vector (dialog)  Indices=6  OutputSizes=1
  x,xdot,xdotdot : Selector  InputPortWidth=18  IndexOptions=Index vector (dialog)  Indices=1  OutputSizes=1
  y,ydot,ydotdot : Selector  InputPortWidth=18  IndexOptions=Index vector (dialog)  Indices=2  OutputSizes=1
  z,zdot,zdotdot : Selector  InputPortWidth=18  IndexOptions=Index vector (dialog)  Indices=3  OutputSizes=1
  SURGE : Outport  VectorParamsAs1DForOutWhenUnconnected=off
  SWAY : Outport  Port=2  VectorParamsAs1DForOutWhenUnconnected=off
  HEAVE : Outport  Port=3  VectorParamsAs1DForOutWhenUnconnected=off
  ROLL : Outport  Port=4  VectorParamsAs1DForOutWhenUnconnected=off
  PITCH : Outport  Port=5  VectorParamsAs1DForOutWhenUnconnected=off
  YAW : Outport  Port=6  VectorParamsAs1DForOutWhenUnconnected=off
  wires:
  x,xdot,xdotdot/1 -> SURGE/1
  y,ydot,ydotdot/1 -> SWAY/1
  z,zdot,zdotdot/1 -> HEAVE/1
  rx,rxdot,rxdotdot/1 -> ROLL/1
  ry,rydot,rydotdot/1 -> PITCH/1
  "rz,rzdot,rzdotdot "/1 -> YAW/1
  6DOF/1 -> rx,rxdot,rxdotdot/1, "rz,rzdot,rzdotdot "/1, ry,rydot,rydotdot/1, y,ydot,ydotdot/1, x,xdot,xdotdot/1, z,zdot,zdotdot/1

== system SM_Offshore_Windturbine/WIND TURBINE/BODIES MOTIONS/Simscape/Blade_1 ==
  Blade : sm_lib/Body Elements/File Solid  ExtGeomFileName=Blade_Default_sldprt.STEP  UnitType=FromFile  ExtGeomFileUnits=m  StepReaderType=HEX  ExportConvexHullGeometry=off  InertiaType=Custom  Mass=smiData.Solid(1).mass  MassUnits=kg  CenterOfMass=smiData.Solid(1).CoM  CenterOfMassUnits=m  MomentsOfInertia=[0 0 0]  MomentsOfInertiaUnits=kg*m^2  ProductsOfInertia=[0 0 0]  ProductsOfInertiaUnits=kg*m^2  BasedOnType=Density  Density=1000  DensityUnits=kg/m^3  DoExposeReferenceFrame=on  SerializedFrames=<Frames/>  GraphicType=FromGeometry  MarkerShape=Sphere  MarkerSize=10  GraphicVisPropType=SimpleVisualProperties  GraphicDiffuseColor=smiData.Solid(1).color  GraphicSpecularColor=[0.5 0.5 0.5 1.0]  GraphicAmbientColor=[0.15 0.15 0.15 1.0]  GraphicEmissiveColor=[0.0 0.0 0.0 1.0]  GraphicShininess=75  GraphicOpacity=smiData.Solid(1).opacity
  ReferenceFrame : sm_lib/Frames and Transforms/Reference Frame
  Transform : sm_lib/Frames and Transforms/Rigid Transform  TranslationMethod=Cartesian  TranslationStandardOffset=0  TranslationLengthUnit=m  TranslationStandardAxis=+Z  TranslationCartesianOffset=smiData.RigidTransform(2).translation  TranslationROffset=0  TranslationROffsetUnits=m  TranslationZOffset=0  TranslationZOffsetUnits=m  TranslationThetaOffset=0  TranslationThetaOffsetUnits=deg  RotationMethod=ArbitraryAxis  RotationAngleUnits=rad  RotationStandardAxis=+Z  RotationAngle=smiData.RigidTransform(2).angle  RotationArbitraryAxis=smiData.RigidTransform(2).axis  FollAlignAxisA=+X  BaseAlignAxisA=+Y  FollAlignAxisB=+Y  BaseAlignAxisB=+Z  RotationSequenceAxes=FollowerAxes  RotationSequence=XYX  RotationSequenceAngles=[0 0 0]  RotationSequenceAnglesUnits=deg  RotationMatrix=[1 0 0; 0 1 0; 0 0 1]
  F : PMIOPort  Side=Left
  connections:
  ReferenceFrame/RConn1 -- Blade/RConn1 -- Transform/LConn1
  Transform/RConn1 -- F/RConn1

== system SM_Offshore_Windturbine/WIND TURBINE/BODIES MOTIONS/Simscape/Blade_2 ==
  Blade : sm_lib/Body Elements/File Solid  ExtGeomFileName=Blade_Default_sldprt.STEP  UnitType=FromFile  ExtGeomFileUnits=m  StepReaderType=HEX  ExportConvexHullGeometry=off  InertiaType=Custom  Mass=smiData.Solid(1).mass  MassUnits=kg  CenterOfMass=smiData.Solid(1).CoM  CenterOfMassUnits=m  MomentsOfInertia=[0 0 0]  MomentsOfInertiaUnits=kg*m^2  ProductsOfInertia=[0 0 0]  ProductsOfInertiaUnits=kg*m^2  BasedOnType=Density  Density=1000  DensityUnits=kg/m^3  DoExposeReferenceFrame=on  SerializedFrames=<Frames/>  GraphicType=FromGeometry  MarkerShape=Sphere  MarkerSize=10  GraphicVisPropType=SimpleVisualProperties  GraphicDiffuseColor=smiData.Solid(1).color  GraphicSpecularColor=[0.5 0.5 0.5 1.0]  GraphicAmbientColor=[0.15 0.15 0.15 1.0]  GraphicEmissiveColor=[0.0 0.0 0.0 1.0]  GraphicShininess=75  GraphicOpacity=smiData.Solid(1).opacity
  ReferenceFrame : sm_lib/Frames and Transforms/Reference Frame
  Transform : sm_lib/Frames and Transforms/Rigid Transform  TranslationMethod=Cartesian  TranslationStandardOffset=0  TranslationLengthUnit=m  TranslationStandardAxis=+Z  TranslationCartesianOffset=smiData.RigidTransform(4).translation  TranslationROffset=0  TranslationROffsetUnits=m  TranslationZOffset=0  TranslationZOffsetUnits=m  TranslationThetaOffset=0  TranslationThetaOffsetUnits=deg  RotationMethod=ArbitraryAxis  RotationAngleUnits=rad  RotationStandardAxis=+Z  RotationAngle=smiData.RigidTransform(4).angle  RotationArbitraryAxis=smiData.RigidTransform(4).axis  FollAlignAxisA=+X  BaseAlignAxisA=+Y  FollAlignAxisB=+Y  BaseAlignAxisB=+Z  RotationSequenceAxes=FollowerAxes  RotationSequence=XYX  RotationSequenceAngles=[0 0 0]  RotationSequenceAnglesUnits=deg  RotationMatrix=[1 0 0; 0 1 0; 0 0 1]
  Transform1 : sm_lib/Frames and Transforms/Rigid Transform  TranslationMethod=Cartesian  TranslationStandardOffset=0  TranslationLengthUnit=m  TranslationStandardAxis=+Z  TranslationCartesianOffset=[0 0 0]  TranslationROffset=0  TranslationROffsetUnits=m  TranslationZOffset=0  TranslationZOffsetUnits=m  TranslationThetaOffset=0  TranslationThetaOffsetUnits=deg  RotationMethod=ArbitraryAxis  RotationAngleUnits=rad  RotationStandardAxis=+Z  RotationAngle=-pi  RotationArbitraryAxis=[0 0 1]  FollAlignAxisA=+X  BaseAlignAxisA=+Y  FollAlignAxisB=+Y  BaseAlignAxisB=+Z  RotationSequenceAxes=FollowerAxes  RotationSequence=XYX  RotationSequenceAngles=[0 0 0]  RotationSequenceAnglesUnits=deg  RotationMatrix=[1 0 0; 0 1 0; 0 0 1]
  F : PMIOPort  Side=Left
  connections:
  ReferenceFrame/RConn1 -- Blade/RConn1 -- Transform/LConn1
  Transform/RConn1 -- Transform1/LConn1
  Transform1/RConn1 -- F/RConn1

== system SM_Offshore_Windturbine/WIND TURBINE/BODIES MOTIONS/Simscape/Blade_3 ==
  Blade : sm_lib/Body Elements/File Solid  ExtGeomFileName=Blade_Default_sldprt.STEP  UnitType=FromFile  ExtGeomFileUnits=m  StepReaderType=HEX  ExportConvexHullGeometry=off  InertiaType=Custom  Mass=smiData.Solid(1).mass  MassUnits=kg  CenterOfMass=smiData.Solid(1).CoM  CenterOfMassUnits=m  MomentsOfInertia=[0 0 0]  MomentsOfInertiaUnits=kg*m^2  ProductsOfInertia=[0 0 0]  ProductsOfInertiaUnits=kg*m^2  BasedOnType=Density  Density=1000  DensityUnits=kg/m^3  DoExposeReferenceFrame=on  SerializedFrames=<Frames/>  GraphicType=FromGeometry  MarkerShape=Sphere  MarkerSize=10  GraphicVisPropType=SimpleVisualProperties  GraphicDiffuseColor=smiData.Solid(1).color  GraphicSpecularColor=[0.5 0.5 0.5 1.0]  GraphicAmbientColor=[0.15 0.15 0.15 1.0]  GraphicEmissiveColor=[0.0 0.0 0.0 1.0]  GraphicShininess=75  GraphicOpacity=smiData.Solid(1).opacity
  ReferenceFrame : sm_lib/Frames and Transforms/Reference Frame
  Transform : sm_lib/Frames and Transforms/Rigid Transform  TranslationMethod=Cartesian  TranslationStandardOffset=0  TranslationLengthUnit=m  TranslationStandardAxis=+Z  TranslationCartesianOffset=smiData.RigidTransform(6).translation  TranslationROffset=0  TranslationROffsetUnits=m  TranslationZOffset=0  TranslationZOffsetUnits=m  TranslationThetaOffset=0  TranslationThetaOffsetUnits=deg  RotationMethod=ArbitraryAxis  RotationAngleUnits=rad  RotationStandardAxis=+Z  RotationAngle=smiData.RigidTransform(6).angle  RotationArbitraryAxis=smiData.RigidTransform(6).axis  FollAlignAxisA=+X  BaseAlignAxisA=+Y  FollAlignAxisB=+Y  BaseAlignAxisB=+Z  RotationSequenceAxes=FollowerAxes  RotationSequence=XYX  RotationSequenceAngles=[0 0 0]  RotationSequenceAnglesUnits=deg  RotationMatrix=[1 0 0; 0 1 0; 0 0 1]
  Transform1 : sm_lib/Frames and Transforms/Rigid Transform  TranslationMethod=Cartesian  TranslationStandardOffset=0  TranslationLengthUnit=m  TranslationStandardAxis=+Z  TranslationCartesianOffset=[0 0 0]  TranslationROffset=0  TranslationROffsetUnits=m  TranslationZOffset=0  TranslationZOffsetUnits=m  TranslationThetaOffset=0  TranslationThetaOffsetUnits=deg  RotationMethod=ArbitraryAxis  RotationAngleUnits=rad  RotationStandardAxis=+Z  RotationAngle=-pi  RotationArbitraryAxis=[0 0 1]  FollAlignAxisA=+X  BaseAlignAxisA=+Y  FollAlignAxisB=+Y  BaseAlignAxisB=+Z  RotationSequenceAxes=FollowerAxes  RotationSequence=XYX  RotationSequenceAngles=[0 0 0]  RotationSequenceAnglesUnits=deg  RotationMatrix=[1 0 0; 0 1 0; 0 0 1]
  F : PMIOPort  Side=Left
  connections:
  ReferenceFrame/RConn1 -- Blade/RConn1 -- Transform/LConn1
  Transform1/RConn1 -- F/RConn1
  Transform/RConn1 -- Transform1/LConn1
